simulink model "mdof_sim"  (R2018b)
settings: Solver=FixedStepAuto  StartTime=0.0  StopTime=Tspan  FixedStep=1e-3  RelTol=1e-3
values from neighbouring files (symbols this model uses):
  A2 = [0 1 0 0 ... (first row only)    [Lab4_Matlab.m]
  amp = 1    [Lab4_Matlab.m]    (also in readfreq2.m = a(minfreq*40+1:maxfreq*40+1,2))
  B2 = [0; 1/m1; 0; 0]    [Lab4_Matlab.m]
  C2 = [1 0 0 0 ... (first row only)    [Lab4_Matlab.m]
  D2 = [0; 0; 0; 0]    [Lab4_Matlab.m]
  freq = 2    [Lab4_Matlab.m]    (also in readfreq2.m = a(minfreq*40+1:maxfreq*40+1,1))
  y0 = [0 0 0 0]    [Lab4_Matlab.m]
settings Model: Creator=Zoe  LastModifiedBy=Zoe

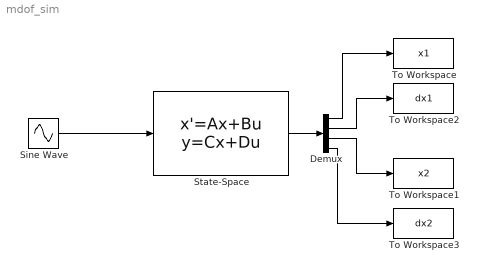
== system mdof_sim ==
  Demux : Demux
  Sine Wave : Sin  Amplitude=amp  Frequency=freq*2*pi  SampleTime=0
  State-Space : StateSpace  A=A2  B=B2  C=C2  D=D2  InitialCondition=y0
  To Workspace : ToWorkspace  VariableName=x1  SaveFormat=Timeseries  SampleTime=-1
  To Workspace1 : ToWorkspace  VariableName=x2  SaveFormat=Timeseries  SampleTime=-1
  To Workspace2 : ToWorkspace  VariableName=dx1  SaveFormat=Timeseries  SampleTime=-1
  To Workspace3 : ToWorkspace  VariableName=dx2  SaveFormat=Timeseries  SampleTime=-1
  wires:
  Sine Wave/1 -> State-Space/1
  State-Space/1 -> Demux/1
  Demux/4 -> To Workspace3/1
  Demux/3 -> To Workspace1/1
  Demux/2 -> To Workspace2/1
  Demux/1 -> To Workspace/1
